simulink model "PI_PSO"  (R2021a)
settings: Solver=VariableStepAuto  StartTime=0.0  StopTime=100  RelTol=1e-6  AbsTol=1e-6
undefined symbols (not defined in the file or in its folder): DiscIntNeverNeededParam, G, Solar_time, wind, wind_time
libraries: powerlib_extras x24, pid_lib x6, simulink x2
(part 1 of 2)
settings Model: Creator=hp  LastModifiedBy=hp
settings SolverCC: ZeroCrossAlgorithm=Adaptive
settings DataIOCC: ReturnWorkspaceOutputs=off
settings DebuggingCC: IgnoredZcDiagnostic=none  SFMachineParentedDataDiag=warning

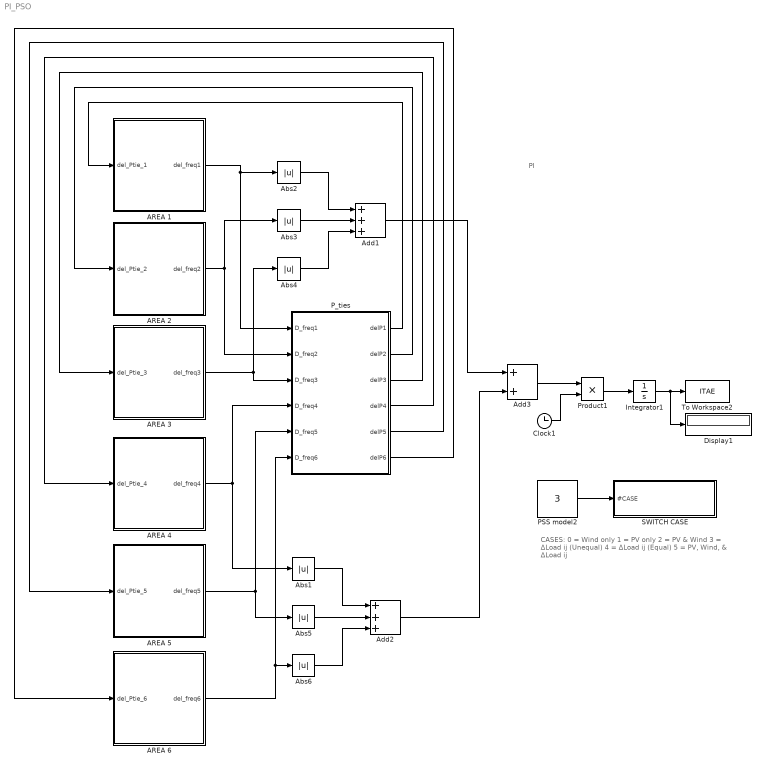
== system PI_PSO ==
  note: PI
  note: CASES:
      |
      | 0 = Wind only
      | 1 = PV only
      | 2 = PV & Wind
      | 3 = ΔLoad ij (Unequal)
      | 4 = ΔLoad ij (Equal)
      | 5 = PV, Wind, & ΔLoad ij
  AREA 1 : Subsystem
  AREA 2 : Subsystem
  AREA 3 : Subsystem
  AREA 4 : Subsystem
  AREA 5 : Subsystem
  AREA 6 : Subsystem
  Abs{1..6} (6 alike) : Abs
  Add1 : Sum  Inputs=+++
  Add2 : Sum  Inputs=+++
  Add3 : Sum
  Clock1 : Clock
  Display1 : Display
  Integrator1 : Integrator
  PSS model2 : Constant  Value=3
  P_ties : Subsystem
  Product1 : Product
  SWITCH CASE : Subsystem
  To Workspace2 : ToWorkspace  VariableName=ITAE  SampleTime=-1
      settings: Save2DSignal=2-D array (concatenate along first dimension)
  wires:
  Abs3/1 -> Add1/2
  AREA 3/1(del_freq3) -> P_ties/3(D_freq3), Abs4/1
  Clock1/1 -> Product1/2
  AREA 1/1(del_freq1) -> P_ties/1(D_freq1), Abs2/1
  AREA 2/1(del_freq2) -> P_ties/2(D_freq2), Abs3/1
  P_ties/2(delP2) -> AREA 2/1(del_Ptie_2)
  Abs4/1 -> Add1/3
  Abs2/1 -> Add1/1
  Add1/1 -> Add3/1
  Product1/1 -> Integrator1/1
  Integrator1/1 -> To Workspace2/1, Display1/1
  P_ties/1(delP1) -> AREA 1/1(del_Ptie_1)
  P_ties/3(delP3) -> AREA 3/1(del_Ptie_3)
  P_ties/4(delP4) -> AREA 4/1(del_Ptie_4)
  P_ties/5(delP5) -> AREA 5/1(del_Ptie_5)
  P_ties/6(delP6) -> AREA 6/1(del_Ptie_6)
  AREA 4/1(del_freq4) -> P_ties/4(D_freq4), Abs1/1
  AREA 5/1(del_freq5) -> P_ties/5(D_freq5), Abs5/1
  AREA 6/1(del_freq6) -> P_ties/6(D_freq6), Abs6/1
  Abs6/1 -> Add2/3
  Abs1/1 -> Add2/1
  Abs5/1 -> Add2/2
  Add2/1 -> Add3/2
  Add3/1 -> Product1/1
  PSS model2/1 -> SWITCH CASE/1(#CASE)

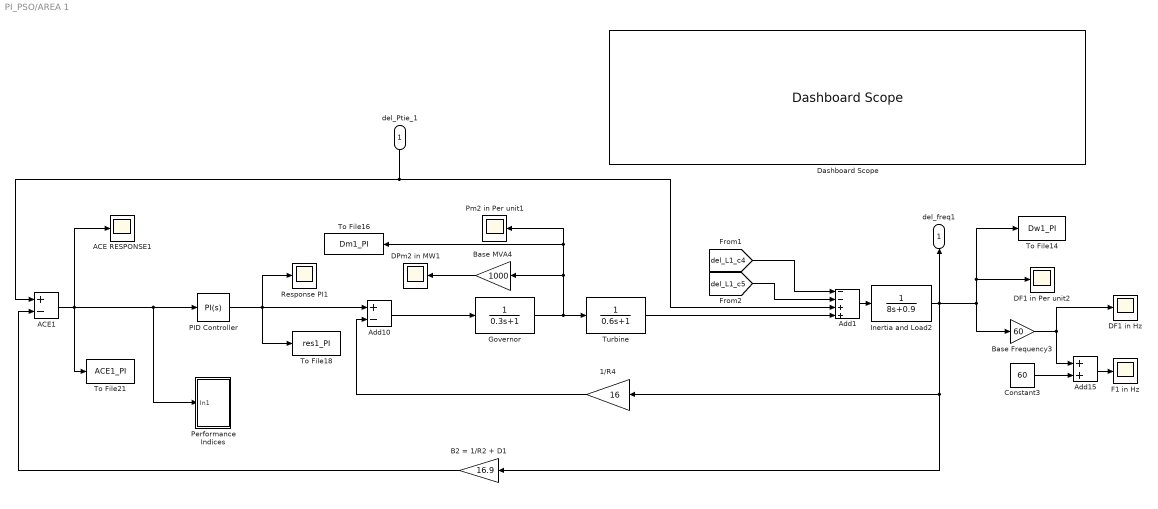
== system PI_PSO/AREA 1 ==
  del_Ptie_1 : Inport
  1/R4 : Gain  Gain=16
  ACE RESPONSE1 : Scope
  ACE1 : Sum  Inputs=+-
  Add1 : Sum  Inputs=--++
  Add10 : Sum  Inputs=+-
  Add15 : Sum
  B2 = 1/R2 + D1 : Gain  Gain=16.9
  Base Frequency3 : Gain  Gain=60
  Base MVA4 : Gain  Gain=1000
  Constant3 : Constant  Value=60
  DF1 in Hz : Scope
  DF1 in Per unit2 : Scope
  DPm2 in MW1 : Scope
  Dashboard Scope : DashboardScope
  F1 in Hz : Scope
  "Governor " : TransferFcn  Denominator=[0.3 1]
  Inertia and Load2 : TransferFcn  Denominator=[8 0.9]
  PID Controller : pid_lib/PID Controller  Controller=PI  Form=Parallel  TimeDomain=Continuous-time  UseExternalTs=off  SampleTime=-1  IntegratorMethod=Forward Euler  FilterMethod=Forward Euler  ControllerParametersSource=internal  P=0.079972086154635  I=0.218754323639510  D=0  UseFilter=on  N=100  TunerSelectOption=Transfer Function Based (PID Tuner App)  InitialConditionSource=internal  InitialConditionForIntegrator=0  InitialConditionForFilter=0  DifferentiatorICPrevScaledInput=0  ExternalReset=none  TrackingMode=off  Kt=1  LimitOutput=off  SatLimitsSource=internal  UpperSaturationLimit=inf  LowerSaturationLimit=-inf  LinearizeAsGain=on  AntiWindupMode=none  Kb=1  POutMin=[]  POutMax=[]  IOutMin=[]  IOutMax=[]  DOutMin=[]  DOutMax=[]  NOutMin=[]  NOutMax=[]  SumOutMin=[]  SumOutMax=[]  SaturationOutMin=[]  SaturationOutMax=[]  PParamMin=[]  PParamMax=[]  IParamMin=[]  IParamMax=[]  DParamMin=[]  DParamMax=[]  NParamMin=[]  NParamMax=[]  KbParamMin=[]  KbParamMax=[]  KtParamMin=[]  KtParamMax=[]  KbOutMin=[]  KbOutMax=[]  KtOutMin=[]  KtOutMax=[]  IntegratorOutMin=[]  IntegratorOutMax=[]  FilterOutMin=[]  FilterOutMax=[]  SumI1OutMin=[]  SumI1OutMax=[]  SumI2OutMin=[]  SumI2OutMax=[]  SumI3OutMin=[]  SumI3OutMax=[]  SumI4OutMin=[]  SumI4OutMax=[]  SumDOutMin=[]  SumDOutMax=[]  DifferentiatorOutMin=[]  DifferentiatorOutMax=[]  FilterDiffOutCoefMin=[]  FilterDiffOutCoefMax=[]  ReciprocalOutMin=[]  ReciprocalOutMax=[]  SumDenOutMin=[]  SumDenOutMax=[]  SumNumOutMin=[]  SumNumOutMax=[]  DivideOutMin=[]  DivideOutMax=[]  UdiffTsProdOutMin=[]  UdiffTsProdOutMax=[]  NTsProdOutMin=[]  NTsProdOutMax=[]  UintegralTsProdOutMin=[]  UintegralTsProdOutMax=[]  UngainTsProdOutMin=[]  UngainTsProdOutMax=[]  IntegratorContinuousStateAttributes=''  IntegratorStateMustResolveToSignalObject=off  IntegratorRTWStateStorageClass=Auto  FilterContinuousStateAttributes=''  FilterStateMustResolveToSignalObject=off  FilterRTWStateStorageClass=Auto  ParallelPVariant=InternalParameters  IdealPVariant=Disabled  IVariant=InternalParameters  DVariant=Disabled  IntegratorVariant=Continuous  SatVariant=Disabled  AWVariant=Passthrough  PCopyVariant=Disabled  TRVariant=Disabled  FdbkBlocksVariant=Forward  IdealPFdbkVariant=Disabled  SatFdbkVariant=Disabled  DerivativeFilterVariant=Disabled  NVariant=Disabled  NCopyVariant=Disabled_SignalSpec  FilterICVariant=Disabled  IntegratorICVariant=InternalICs  ExternalResetVariant=Disabled  TRSumVariant=Passthrough  SumFdbkVariant=Disabled  SumVariant=Sum_PI  TsampFilterVariant=InternalTs  TsampNgainVariant=Passthrough  TsampIntegralVariant=Passthrough  ExternalSaturationOutDataTypeStr=Inherit: Same as second input
  Performance Indices : Subsystem
  Pm2 in Per unit1 : Scope
  Response PI1 : Scope
  To File14 : ToFile  Filename=Dw1_PI  MatrixName=Dw1_PI
  To File16 : ToFile  Filename=Dm1_PI  MatrixName=Dm1_PI
  To File18 : ToFile  Filename=res1_PI  MatrixName=res1_PI
  To File21 : ToFile  Filename=ACE1_PI  MatrixName=ACE1_PI
  Turbine : TransferFcn  Denominator=[0.6 1]
  del_freq1 : Outport
  wires:
  PID Controller/1 -> Response PI1/1, Add10/1, To File18/1
  1/R4/1 -> Add10/2
  Base MVA4/1 -> DPm2 in MW1/1
  Constant3/1 -> Add15/2
  Add15/1 -> F1 in Hz/1
  Base Frequency3/1 -> DF1 in Hz/1, Add15/1
  B2 = 1/R2 + D1/1 -> ACE1/2
  del_Ptie_1/1 -> Add1/3, ACE1/1
  Inertia and Load2/1 -> Base Frequency3/1, To File14/1, DF1 in Per unit2/1, 1/R4/1, B2 = 1/R2 + D1/1, del_freq1/1
  Add1/1 -> Inertia and Load2/1
  ACE1/1 -> PID Controller/1, Performance Indices/1(In1), To File21/1, ACE RESPONSE1/1
  Turbine/1 -> Add1/4
  [del_L1_c4] -> Add1/1
  [del_L1_c5] -> Add1/2
  "Governor "/1 -> Turbine/1, Pm2 in Per unit1/1, To File16/1, Base MVA4/1
  Add10/1 -> "Governor "/1

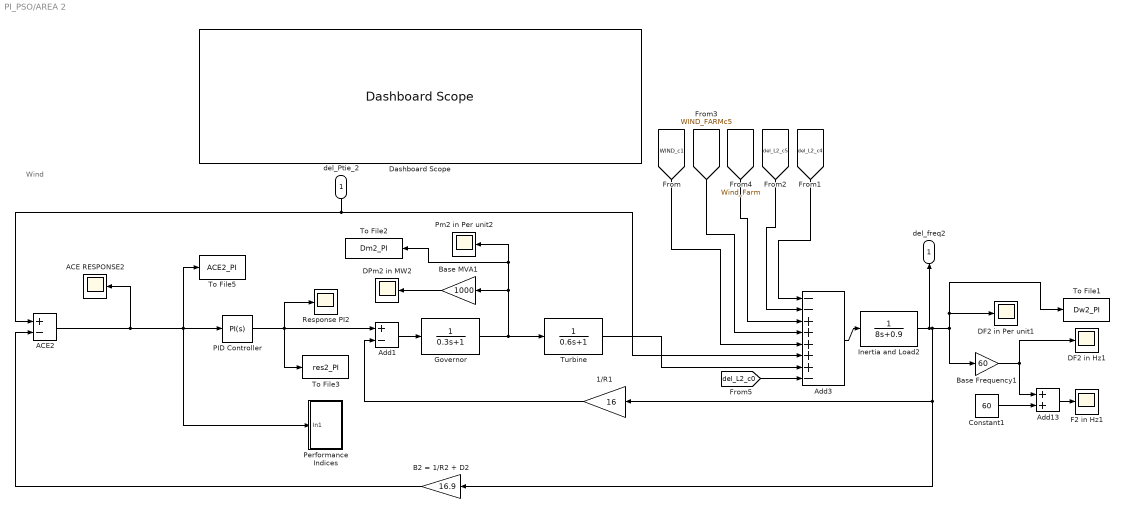
== system PI_PSO/AREA 2 ==
  note: Wind
  del_Ptie_2 : Inport
  1/R1 : Gain  Gain=16
  ACE RESPONSE2 : Scope
  ACE2 : Sum  Inputs=+-
  Add1 : Sum  Inputs=+-
  Add13 : Sum
  Add3 : Sum  Inputs=--+++++-
  B2 = 1/R2 + D2 : Gain  Gain=16.9
  Base Frequency1 : Gain  Gain=60
  Base MVA1 : Gain  Gain=1000
  Constant1 : Constant  Value=60
  DF2 in Hz1 : Scope
  DF2 in Per unit1 : Scope
  DPm2 in MW2 : Scope
  Dashboard Scope : DashboardScope
  F2 in Hz1 : Scope
  "Governor " : TransferFcn  Denominator=[0.3 1]
  Inertia and Load2 : TransferFcn  Denominator=[8 0.9]
  PID Controller : pid_lib/PID Controller  Controller=PI  Form=Parallel  TimeDomain=Continuous-time  UseExternalTs=off  SampleTime=-1  IntegratorMethod=Forward Euler  FilterMethod=Forward Euler  ControllerParametersSource=internal  P=-0.193992496547051  I=0.445472440969199  D=0  UseFilter=on  N=100  TunerSelectOption=Transfer Function Based (PID Tuner App)  InitialConditionSource=internal  InitialConditionForIntegrator=0  InitialConditionForFilter=0  DifferentiatorICPrevScaledInput=0  ExternalReset=none  TrackingMode=off  Kt=1  LimitOutput=off  SatLimitsSource=internal  UpperSaturationLimit=inf  LowerSaturationLimit=-inf  LinearizeAsGain=on  AntiWindupMode=none  Kb=1  POutMin=[]  POutMax=[]  IOutMin=[]  IOutMax=[]  DOutMin=[]  DOutMax=[]  NOutMin=[]  NOutMax=[]  SumOutMin=[]  SumOutMax=[]  SaturationOutMin=[]  SaturationOutMax=[]  PParamMin=[]  PParamMax=[]  IParamMin=[]  IParamMax=[]  DParamMin=[]  DParamMax=[]  NParamMin=[]  NParamMax=[]  KbParamMin=[]  KbParamMax=[]  KtParamMin=[]  KtParamMax=[]  KbOutMin=[]  KbOutMax=[]  KtOutMin=[]  KtOutMax=[]  IntegratorOutMin=[]  IntegratorOutMax=[]  FilterOutMin=[]  FilterOutMax=[]  SumI1OutMin=[]  SumI1OutMax=[]  SumI2OutMin=[]  SumI2OutMax=[]  SumI3OutMin=[]  SumI3OutMax=[]  SumI4OutMin=[]  SumI4OutMax=[]  SumDOutMin=[]  SumDOutMax=[]  DifferentiatorOutMin=[]  DifferentiatorOutMax=[]  FilterDiffOutCoefMin=[]  FilterDiffOutCoefMax=[]  ReciprocalOutMin=[]  ReciprocalOutMax=[]  SumDenOutMin=[]  SumDenOutMax=[]  SumNumOutMin=[]  SumNumOutMax=[]  DivideOutMin=[]  DivideOutMax=[]  UdiffTsProdOutMin=[]  UdiffTsProdOutMax=[]  NTsProdOutMin=[]  NTsProdOutMax=[]  UintegralTsProdOutMin=[]  UintegralTsProdOutMax=[]  UngainTsProdOutMin=[]  UngainTsProdOutMax=[]  IntegratorContinuousStateAttributes=''  IntegratorStateMustResolveToSignalObject=off  IntegratorRTWStateStorageClass=Auto  FilterContinuousStateAttributes=''  FilterStateMustResolveToSignalObject=off  FilterRTWStateStorageClass=Auto  ParallelPVariant=InternalParameters  IdealPVariant=Disabled  IVariant=InternalParameters  DVariant=Disabled  IntegratorVariant=Continuous  SatVariant=Disabled  AWVariant=Passthrough  PCopyVariant=Disabled  TRVariant=Disabled  FdbkBlocksVariant=Forward  IdealPFdbkVariant=Disabled  SatFdbkVariant=Disabled  DerivativeFilterVariant=Disabled  NVariant=Disabled  NCopyVariant=Disabled_SignalSpec  FilterICVariant=Disabled  IntegratorICVariant=InternalICs  ExternalResetVariant=Disabled  TRSumVariant=Passthrough  SumFdbkVariant=Disabled  SumVariant=Sum_PI  TsampFilterVariant=InternalTs  TsampNgainVariant=Passthrough  TsampIntegralVariant=Passthrough  ExternalSaturationOutDataTypeStr=Inherit: Same as second input
  Performance Indices : Subsystem
  Pm2 in Per unit2 : Scope
  Response PI2 : Scope
  To File1 : ToFile  Filename=Dw2_PI  MatrixName=Dw2_PI
  To File2 : ToFile  Filename=Dm2_PI  MatrixName=Dm2_PI
  To File3 : ToFile  Filename=res2_PI  MatrixName=res2_PI
  To File5 : ToFile  Filename=ACE2_PI  MatrixName=ACE2_PI
  Turbine : TransferFcn  Denominator=[0.6 1]
  del_freq2 : Outport
  wires:
  del_Ptie_2/1 -> Add3/6, ACE2/1
  Inertia and Load2/1 -> Base Frequency1/1, To File1/1, DF2 in Per unit1/1, 1/R1/1, B2 = 1/R2 + D2/1, del_freq2/1
  Add13/1 -> F2 in Hz1/1
  Add3/1 -> Inertia and Load2/1
  1/R1/1 -> Add1/2
  Base Frequency1/1 -> DF2 in Hz1/1, Add13/1
  Base MVA1/1 -> DPm2 in MW2/1
  B2 = 1/R2 + D2/1 -> ACE2/2
  PID Controller/1 -> To File3/1, Response PI2/1, Add1/1
  Constant1/1 -> Add13/2
  ACE2/1 -> ACE RESPONSE2/1, PID Controller/1, Performance Indices/1(In1), To File5/1
  Turbine/1 -> Add3/7
  [WIND_c1] -> Add3/5
  [WIND_FARMc5] -> Add3/4
  [Wind_Farm] -> Add3/3
  [del_L2_c5] -> Add3/2
  [del_L2_c4] -> Add3/1
  "Governor "/1 -> Turbine/1, Pm2 in Per unit2/1, To File2/1, Base MVA1/1
  Add1/1 -> "Governor "/1
  [del_L2_c0] -> Add3/8

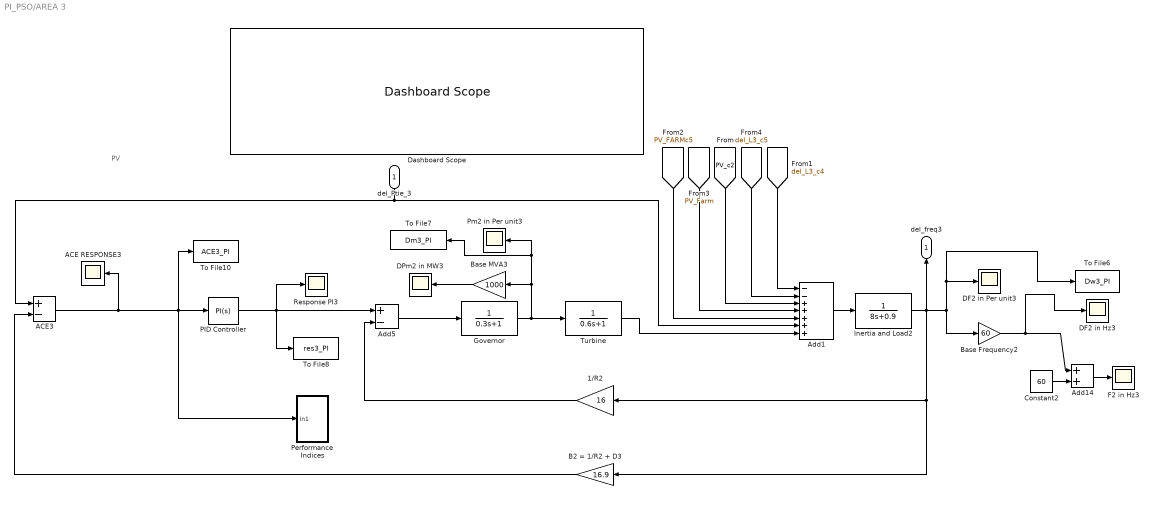
== system PI_PSO/AREA 3 ==
  note: PV
  del_Ptie_3 : Inport
  1/R2 : Gain  Gain=16
  ACE RESPONSE3 : Scope
  ACE3 : Sum  Inputs=+-
  Add1 : Sum  Inputs=--+++++
  Add14 : Sum
  Add5 : Sum  Inputs=+-
  B2 = 1/R2 + D3 : Gain  Gain=16.9
  Base Frequency2 : Gain  Gain=60
  Base MVA3 : Gain  Gain=1000
  Constant2 : Constant  Value=60
  DF2 in Hz3 : Scope
  DF2 in Per unit3 : Scope
  DPm2 in MW3 : Scope
  Dashboard Scope : DashboardScope
  F2 in Hz3 : Scope
  "Governor " : TransferFcn  Denominator=[0.3 1]
  Inertia and Load2 : TransferFcn  Denominator=[8 0.9]
  PID Controller : pid_lib/PID Controller  Controller=PI  Form=Parallel  TimeDomain=Continuous-time  UseExternalTs=off  SampleTime=-1  IntegratorMethod=Forward Euler  FilterMethod=Forward Euler  ControllerParametersSource=internal  P=-0.208794341045674  I=0.479449973673102  D=0  UseFilter=on  N=100  TunerSelectOption=Transfer Function Based (PID Tuner App)  InitialConditionSource=internal  InitialConditionForIntegrator=0  InitialConditionForFilter=0  DifferentiatorICPrevScaledInput=0  ExternalReset=none  TrackingMode=off  Kt=1  LimitOutput=off  SatLimitsSource=internal  UpperSaturationLimit=inf  LowerSaturationLimit=-inf  LinearizeAsGain=on  AntiWindupMode=none  Kb=1  POutMin=[]  POutMax=[]  IOutMin=[]  IOutMax=[]  DOutMin=[]  DOutMax=[]  NOutMin=[]  NOutMax=[]  SumOutMin=[]  SumOutMax=[]  SaturationOutMin=[]  SaturationOutMax=[]  PParamMin=[]  PParamMax=[]  IParamMin=[]  IParamMax=[]  DParamMin=[]  DParamMax=[]  NParamMin=[]  NParamMax=[]  KbParamMin=[]  KbParamMax=[]  KtParamMin=[]  KtParamMax=[]  KbOutMin=[]  KbOutMax=[]  KtOutMin=[]  KtOutMax=[]  IntegratorOutMin=[]  IntegratorOutMax=[]  FilterOutMin=[]  FilterOutMax=[]  SumI1OutMin=[]  SumI1OutMax=[]  SumI2OutMin=[]  SumI2OutMax=[]  SumI3OutMin=[]  SumI3OutMax=[]  SumI4OutMin=[]  SumI4OutMax=[]  SumDOutMin=[]  SumDOutMax=[]  DifferentiatorOutMin=[]  DifferentiatorOutMax=[]  FilterDiffOutCoefMin=[]  FilterDiffOutCoefMax=[]  ReciprocalOutMin=[]  ReciprocalOutMax=[]  SumDenOutMin=[]  SumDenOutMax=[]  SumNumOutMin=[]  SumNumOutMax=[]  DivideOutMin=[]  DivideOutMax=[]  UdiffTsProdOutMin=[]  UdiffTsProdOutMax=[]  NTsProdOutMin=[]  NTsProdOutMax=[]  UintegralTsProdOutMin=[]  UintegralTsProdOutMax=[]  UngainTsProdOutMin=[]  UngainTsProdOutMax=[]  IntegratorContinuousStateAttributes=''  IntegratorStateMustResolveToSignalObject=off  IntegratorRTWStateStorageClass=Auto  FilterContinuousStateAttributes=''  FilterStateMustResolveToSignalObject=off  FilterRTWStateStorageClass=Auto  ParallelPVariant=InternalParameters  IdealPVariant=Disabled  IVariant=InternalParameters  DVariant=Disabled  IntegratorVariant=Continuous  SatVariant=Disabled  AWVariant=Passthrough  PCopyVariant=Disabled  TRVariant=Disabled  FdbkBlocksVariant=Forward  IdealPFdbkVariant=Disabled  SatFdbkVariant=Disabled  DerivativeFilterVariant=Disabled  NVariant=Disabled  NCopyVariant=Disabled_SignalSpec  FilterICVariant=Disabled  IntegratorICVariant=InternalICs  ExternalResetVariant=Disabled  TRSumVariant=Passthrough  SumFdbkVariant=Disabled  SumVariant=Sum_PI  TsampFilterVariant=InternalTs  TsampNgainVariant=Passthrough  TsampIntegralVariant=Passthrough  ExternalSaturationOutDataTypeStr=Inherit: Same as second input
  Performance Indices : Subsystem
  Pm2 in Per unit3 : Scope
  Response PI3 : Scope
  To File10 : ToFile  Filename=ACE3_PI  MatrixName=ACE3_PI
  To File6 : ToFile  Filename=Dw3_PI  MatrixName=Dw3_PI
  To File7 : ToFile  Filename=Dm3_PI  MatrixName=Dm3_PI
  To File8 : ToFile  Filename=res3_PI  MatrixName=res3_PI
  Turbine : TransferFcn  Denominator=[0.6 1]
  del_freq3 : Outport
  wires:
  PID Controller/1 -> To File8/1, Response PI3/1, Add5/1
  Constant2/1 -> Add14/2
  Base MVA3/1 -> DPm2 in MW3/1
  1/R2/1 -> Add5/2
  Base Frequency2/1 -> Add14/1, DF2 in Hz3/1
  Add14/1 -> F2 in Hz3/1
  del_Ptie_3/1 -> ACE3/1, Add1/6
  B2 = 1/R2 + D3/1 -> ACE3/2
  Add1/1 -> Inertia and Load2/1
  Inertia and Load2/1 -> 1/R2/1, B2 = 1/R2 + D3/1, Base Frequency2/1, To File6/1, DF2 in Per unit3/1, del_freq3/1
  ACE3/1 -> ACE RESPONSE3/1, PID Controller/1, Performance Indices/1(In1), To File10/1
  Turbine/1 -> Add1/7
  [PV_FARMc5] -> Add1/5
  [PV_Farm] -> Add1/4
  [PV_c2] -> Add1/3
  [del_L3_c5] -> Add1/2
  [del_L3_c4] -> Add1/1
  Add5/1 -> "Governor "/1
  "Governor "/1 -> Turbine/1, To File7/1, Pm2 in Per unit3/1, Base MVA3/1

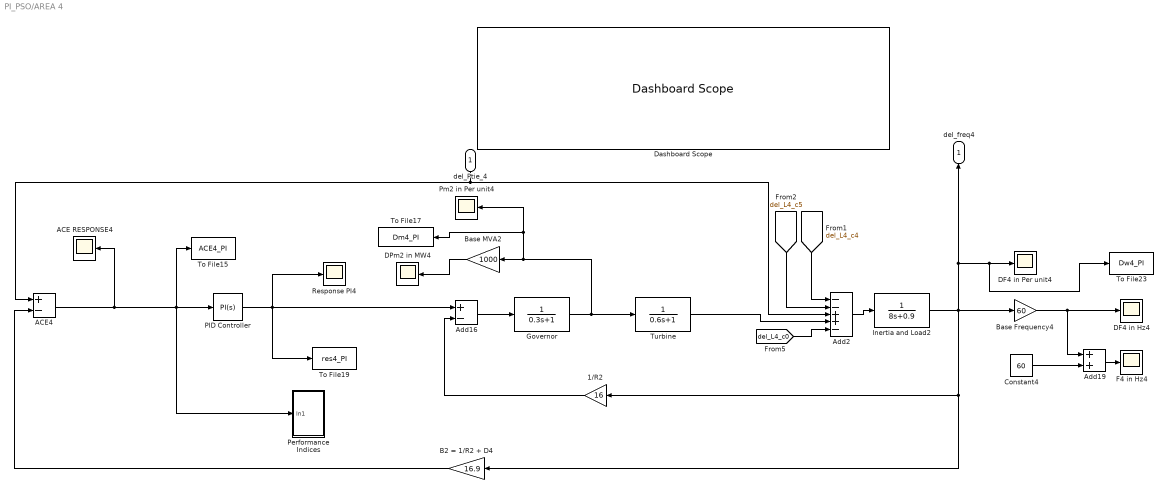
== system PI_PSO/AREA 4 ==
  del_Ptie_4 : Inport
  1/R2 : Gain  Gain=16
  ACE RESPONSE4 : Scope
  ACE4 : Sum  Inputs=+-
  Add16 : Sum  Inputs=+-
  Add19 : Sum
  Add2 : Sum  Inputs=--++-
  B2 = 1/R2 + D4 : Gain  Gain=16.9
  Base Frequency4 : Gain  Gain=60
  Base MVA2 : Gain  Gain=1000
  Constant4 : Constant  Value=60
  DF4 in Hz4 : Scope
  DF4 in Per unit4 : Scope
  DPm2 in MW4 : Scope
  Dashboard Scope : DashboardScope
  F4 in Hz4 : Scope
  "Governor " : TransferFcn  Denominator=[0.3 1]
  Inertia and Load2 : TransferFcn  Denominator=[8 0.9]
  PID Controller : pid_lib/PID Controller  Controller=PI  Form=Parallel  TimeDomain=Continuous-time  UseExternalTs=off  SampleTime=-1  IntegratorMethod=Forward Euler  FilterMethod=Forward Euler  ControllerParametersSource=internal  P=0.085231271598390  I=0.194395137959333  D=0  UseFilter=on  N=100  TunerSelectOption=Transfer Function Based (PID Tuner App)  InitialConditionSource=internal  InitialConditionForIntegrator=0  InitialConditionForFilter=0  DifferentiatorICPrevScaledInput=0  ExternalReset=none  TrackingMode=off  Kt=1  LimitOutput=off  SatLimitsSource=internal  UpperSaturationLimit=inf  LowerSaturationLimit=-inf  LinearizeAsGain=on  AntiWindupMode=none  Kb=1  POutMin=[]  POutMax=[]  IOutMin=[]  IOutMax=[]  DOutMin=[]  DOutMax=[]  NOutMin=[]  NOutMax=[]  SumOutMin=[]  SumOutMax=[]  SaturationOutMin=[]  SaturationOutMax=[]  PParamMin=[]  PParamMax=[]  IParamMin=[]  IParamMax=[]  DParamMin=[]  DParamMax=[]  NParamMin=[]  NParamMax=[]  KbParamMin=[]  KbParamMax=[]  KtParamMin=[]  KtParamMax=[]  KbOutMin=[]  KbOutMax=[]  KtOutMin=[]  KtOutMax=[]  IntegratorOutMin=[]  IntegratorOutMax=[]  FilterOutMin=[]  FilterOutMax=[]  SumI1OutMin=[]  SumI1OutMax=[]  SumI2OutMin=[]  SumI2OutMax=[]  SumI3OutMin=[]  SumI3OutMax=[]  SumI4OutMin=[]  SumI4OutMax=[]  SumDOutMin=[]  SumDOutMax=[]  DifferentiatorOutMin=[]  DifferentiatorOutMax=[]  FilterDiffOutCoefMin=[]  FilterDiffOutCoefMax=[]  ReciprocalOutMin=[]  ReciprocalOutMax=[]  SumDenOutMin=[]  SumDenOutMax=[]  SumNumOutMin=[]  SumNumOutMax=[]  DivideOutMin=[]  DivideOutMax=[]  UdiffTsProdOutMin=[]  UdiffTsProdOutMax=[]  NTsProdOutMin=[]  NTsProdOutMax=[]  UintegralTsProdOutMin=[]  UintegralTsProdOutMax=[]  UngainTsProdOutMin=[]  UngainTsProdOutMax=[]  IntegratorContinuousStateAttributes=''  IntegratorStateMustResolveToSignalObject=off  IntegratorRTWStateStorageClass=Auto  FilterContinuousStateAttributes=''  FilterStateMustResolveToSignalObject=off  FilterRTWStateStorageClass=Auto  ParallelPVariant=InternalParameters  IdealPVariant=Disabled  IVariant=InternalParameters  DVariant=Disabled  IntegratorVariant=Continuous  SatVariant=Disabled  AWVariant=Passthrough  PCopyVariant=Disabled  TRVariant=Disabled  FdbkBlocksVariant=Forward  IdealPFdbkVariant=Disabled  SatFdbkVariant=Disabled  DerivativeFilterVariant=Disabled  NVariant=Disabled  NCopyVariant=Disabled_SignalSpec  FilterICVariant=Disabled  IntegratorICVariant=InternalICs  ExternalResetVariant=Disabled  TRSumVariant=Passthrough  SumFdbkVariant=Disabled  SumVariant=Sum_PI  TsampFilterVariant=InternalTs  TsampNgainVariant=Passthrough  TsampIntegralVariant=Passthrough  ExternalSaturationOutDataTypeStr=Inherit: Same as second input
  Performance Indices : Subsystem
  Pm2 in Per unit4 : Scope
  Response PI4 : Scope
  To File15 : ToFile  Filename=ACE4_PI  MatrixName=ACE4_PI
  To File17 : ToFile  Filename=Dm4_PI  MatrixName=Dm4_PI
  To File19 : ToFile  Filename=res4_PI  MatrixName=res4_PI
  To File23 : ToFile  Filename=Dw4_PI  MatrixName=Dw4_PI
  Turbine : TransferFcn  Denominator=[0.6 1]
  del_freq4 : Outport
  wires:
  ACE4/1 -> ACE RESPONSE4/1, PID Controller/1, Performance Indices/1(In1), To File15/1
  Constant4/1 -> Add19/2
  Add2/1 -> Inertia and Load2/1
  Add19/1 -> F4 in Hz4/1
  B2 = 1/R2 + D4/1 -> ACE4/2
  Base MVA2/1 -> DPm2 in MW4/1
  Inertia and Load2/1 -> B2 = 1/R2 + D4/1, 1/R2/1, Base Frequency4/1, del_freq4/1, To File23/1, DF4 in Per unit4/1
  Base Frequency4/1 -> DF4 in Hz4/1, Add19/1
  1/R2/1 -> Add16/2
  del_Ptie_4/1 -> Add2/3, ACE4/1
  [del_L4_c5] -> Add2/2
  [del_L4_c4] -> Add2/1
  PID Controller/1 -> To File19/1, Response PI4/1, Add16/1
  Add16/1 -> "Governor "/1
  "Governor "/1 -> Turbine/1, To File17/1, Pm2 in Per unit4/1, Base MVA2/1
  Turbine/1 -> Add2/4
  [del_L4_c0] -> Add2/5

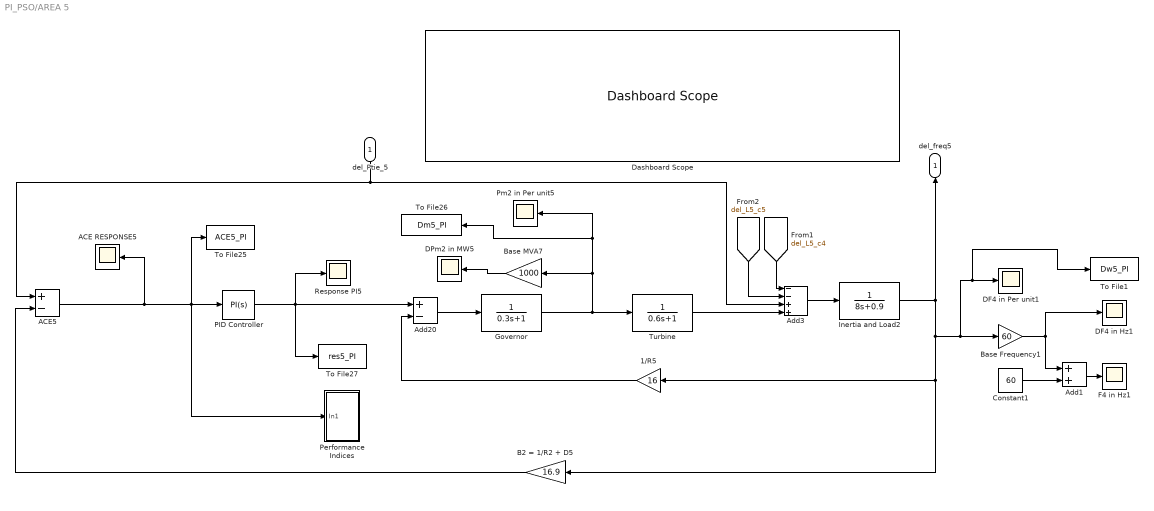
== system PI_PSO/AREA 5 ==
  del_Ptie_5 : Inport
  1/R5 : Gain  Gain=16
  ACE RESPONSE5 : Scope
  ACE5 : Sum  Inputs=+-
  Add1 : Sum
  Add20 : Sum  Inputs=+-
  Add3 : Sum  Inputs=--++
  B2 = 1/R2 + D5 : Gain  Gain=16.9
  Base Frequency1 : Gain  Gain=60
  Base MVA7 : Gain  Gain=1000
  Constant1 : Constant  Value=60
  DF4 in Hz1 : Scope
  DF4 in Per unit1 : Scope
  DPm2 in MW5 : Scope
  Dashboard Scope : DashboardScope
  F4 in Hz1 : Scope
  "Governor " : TransferFcn  Denominator=[0.3 1]
  Inertia and Load2 : TransferFcn  Denominator=[8 0.9]
  PID Controller : pid_lib/PID Controller  Controller=PI  Form=Parallel  TimeDomain=Continuous-time  UseExternalTs=off  SampleTime=-1  IntegratorMethod=Forward Euler  FilterMethod=Forward Euler  ControllerParametersSource=internal  P=-0.426469161483215  I=0.210966324969466  D=0  UseFilter=on  N=100  TunerSelectOption=Transfer Function Based (PID Tuner App)  InitialConditionSource=internal  InitialConditionForIntegrator=0  InitialConditionForFilter=0  DifferentiatorICPrevScaledInput=0  ExternalReset=none  TrackingMode=off  Kt=1  LimitOutput=off  SatLimitsSource=internal  UpperSaturationLimit=inf  LowerSaturationLimit=-inf  LinearizeAsGain=on  AntiWindupMode=none  Kb=1  POutMin=[]  POutMax=[]  IOutMin=[]  IOutMax=[]  DOutMin=[]  DOutMax=[]  NOutMin=[]  NOutMax=[]  SumOutMin=[]  SumOutMax=[]  SaturationOutMin=[]  SaturationOutMax=[]  PParamMin=[]  PParamMax=[]  IParamMin=[]  IParamMax=[]  DParamMin=[]  DParamMax=[]  NParamMin=[]  NParamMax=[]  KbParamMin=[]  KbParamMax=[]  KtParamMin=[]  KtParamMax=[]  KbOutMin=[]  KbOutMax=[]  KtOutMin=[]  KtOutMax=[]  IntegratorOutMin=[]  IntegratorOutMax=[]  FilterOutMin=[]  FilterOutMax=[]  SumI1OutMin=[]  SumI1OutMax=[]  SumI2OutMin=[]  SumI2OutMax=[]  SumI3OutMin=[]  SumI3OutMax=[]  SumI4OutMin=[]  SumI4OutMax=[]  SumDOutMin=[]  SumDOutMax=[]  DifferentiatorOutMin=[]  DifferentiatorOutMax=[]  FilterDiffOutCoefMin=[]  FilterDiffOutCoefMax=[]  ReciprocalOutMin=[]  ReciprocalOutMax=[]  SumDenOutMin=[]  SumDenOutMax=[]  SumNumOutMin=[]  SumNumOutMax=[]  DivideOutMin=[]  DivideOutMax=[]  UdiffTsProdOutMin=[]  UdiffTsProdOutMax=[]  NTsProdOutMin=[]  NTsProdOutMax=[]  UintegralTsProdOutMin=[]  UintegralTsProdOutMax=[]  UngainTsProdOutMin=[]  UngainTsProdOutMax=[]  IntegratorContinuousStateAttributes=''  IntegratorStateMustResolveToSignalObject=off  IntegratorRTWStateStorageClass=Auto  FilterContinuousStateAttributes=''  FilterStateMustResolveToSignalObject=off  FilterRTWStateStorageClass=Auto  ParallelPVariant=InternalParameters  IdealPVariant=Disabled  IVariant=InternalParameters  DVariant=Disabled  IntegratorVariant=Continuous  SatVariant=Disabled  AWVariant=Passthrough  PCopyVariant=Disabled  TRVariant=Disabled  FdbkBlocksVariant=Forward  IdealPFdbkVariant=Disabled  SatFdbkVariant=Disabled  DerivativeFilterVariant=Disabled  NVariant=Disabled  NCopyVariant=Disabled_SignalSpec  FilterICVariant=Disabled  IntegratorICVariant=InternalICs  ExternalResetVariant=Disabled  TRSumVariant=Passthrough  SumFdbkVariant=Disabled  SumVariant=Sum_PI  TsampFilterVariant=InternalTs  TsampNgainVariant=Passthrough  TsampIntegralVariant=Passthrough  ExternalSaturationOutDataTypeStr=Inherit: Same as second input
  Performance Indices : Subsystem
  Pm2 in Per unit5 : Scope
  Response PI5 : Scope
  To File1 : ToFile  Filename=Dw5_PI  MatrixName=Dw5_PI
  To File25 : ToFile  Filename=ACE5_PI  MatrixName=ACE5_PI
  To File26 : ToFile  Filename=Dm5_PI  MatrixName=Dm5_PI
  To File27 : ToFile  Filename=res5_PI  MatrixName=res5_PI
  Turbine : TransferFcn  Denominator=[0.6 1]
  del_freq5 : Outport
  wires:
  Constant1/1 -> Add1/2
  Base MVA7/1 -> DPm2 in MW5/1
  Base Frequency1/1 -> DF4 in Hz1/1, Add1/1
  Add1/1 -> F4 in Hz1/1
  1/R5/1 -> Add20/2
  Add3/1 -> Inertia and Load2/1
  ACE5/1 -> ACE RESPONSE5/1, PID Controller/1, Performance Indices/1(In1), To File25/1
  B2 = 1/R2 + D5/1 -> ACE5/2
  Inertia and Load2/1 -> B2 = 1/R2 + D5/1, 1/R5/1, To File1/1, DF4 in Per unit1/1, Base Frequency1/1, del_freq5/1
  Turbine/1 -> Add3/4
  del_Ptie_5/1 -> ACE5/1, Add3/3
  [del_L5_c5] -> Add3/2
  [del_L5_c4] -> Add3/1
  PID Controller/1 -> To File27/1, Add20/1, Response PI5/1
  Add20/1 -> "Governor "/1
  "Governor "/1 -> To File26/1, Pm2 in Per unit5/1, Base MVA7/1, Turbine/1

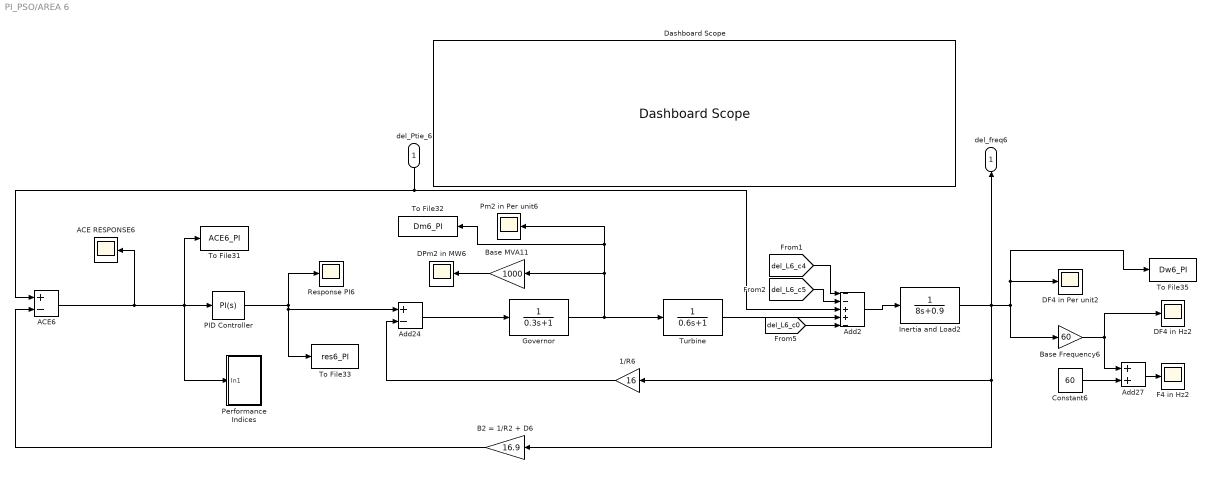
== system PI_PSO/AREA 6 ==
  del_Ptie_6 : Inport
  1/R6 : Gain  Gain=16
  ACE RESPONSE6 : Scope
  ACE6 : Sum  Inputs=+-
  Add2 : Sum  Inputs=--++-
  Add24 : Sum  Inputs=+-
  Add27 : Sum
  B2 = 1/R2 + D6 : Gain  Gain=16.9
  Base Frequency6 : Gain  Gain=60
  Base MVA11 : Gain  Gain=1000
  Constant6 : Constant  Value=60
  DF4 in Hz2 : Scope
  DF4 in Per unit2 : Scope
  DPm2 in MW6 : Scope
  Dashboard Scope : DashboardScope
  F4 in Hz2 : Scope
  "Governor " : TransferFcn  Denominator=[0.3 1]
  Inertia and Load2 : TransferFcn  Denominator=[8 0.9]
  PID Controller : pid_lib/PID Controller  Controller=PI  Form=Parallel  TimeDomain=Continuous-time  UseExternalTs=off  SampleTime=-1  IntegratorMethod=Forward Euler  FilterMethod=Forward Euler  ControllerParametersSource=internal  P=-0.029658962972710  I=0.090847703671048  D=0  UseFilter=on  N=100  TunerSelectOption=Transfer Function Based (PID Tuner App)  InitialConditionSource=internal  InitialConditionForIntegrator=0  InitialConditionForFilter=0  DifferentiatorICPrevScaledInput=0  ExternalReset=none  TrackingMode=off  Kt=1  LimitOutput=off  SatLimitsSource=internal  UpperSaturationLimit=inf  LowerSaturationLimit=-inf  LinearizeAsGain=on  AntiWindupMode=none  Kb=1  POutMin=[]  POutMax=[]  IOutMin=[]  IOutMax=[]  DOutMin=[]  DOutMax=[]  NOutMin=[]  NOutMax=[]  SumOutMin=[]  SumOutMax=[]  SaturationOutMin=[]  SaturationOutMax=[]  PParamMin=[]  PParamMax=[]  IParamMin=[]  IParamMax=[]  DParamMin=[]  DParamMax=[]  NParamMin=[]  NParamMax=[]  KbParamMin=[]  KbParamMax=[]  KtParamMin=[]  KtParamMax=[]  KbOutMin=[]  KbOutMax=[]  KtOutMin=[]  KtOutMax=[]  IntegratorOutMin=[]  IntegratorOutMax=[]  FilterOutMin=[]  FilterOutMax=[]  SumI1OutMin=[]  SumI1OutMax=[]  SumI2OutMin=[]  SumI2OutMax=[]  SumI3OutMin=[]  SumI3OutMax=[]  SumI4OutMin=[]  SumI4OutMax=[]  SumDOutMin=[]  SumDOutMax=[]  DifferentiatorOutMin=[]  DifferentiatorOutMax=[]  FilterDiffOutCoefMin=[]  FilterDiffOutCoefMax=[]  ReciprocalOutMin=[]  ReciprocalOutMax=[]  SumDenOutMin=[]  SumDenOutMax=[]  SumNumOutMin=[]  SumNumOutMax=[]  DivideOutMin=[]  DivideOutMax=[]  UdiffTsProdOutMin=[]  UdiffTsProdOutMax=[]  NTsProdOutMin=[]  NTsProdOutMax=[]  UintegralTsProdOutMin=[]  UintegralTsProdOutMax=[]  UngainTsProdOutMin=[]  UngainTsProdOutMax=[]  IntegratorContinuousStateAttributes=''  IntegratorStateMustResolveToSignalObject=off  IntegratorRTWStateStorageClass=Auto  FilterContinuousStateAttributes=''  FilterStateMustResolveToSignalObject=off  FilterRTWStateStorageClass=Auto  ParallelPVariant=InternalParameters  IdealPVariant=Disabled  IVariant=InternalParameters  DVariant=Disabled  IntegratorVariant=Continuous  SatVariant=Disabled  AWVariant=Passthrough  PCopyVariant=Disabled  TRVariant=Disabled  FdbkBlocksVariant=Forward  IdealPFdbkVariant=Disabled  SatFdbkVariant=Disabled  DerivativeFilterVariant=Disabled  NVariant=Disabled  NCopyVariant=Disabled_SignalSpec  FilterICVariant=Disabled  IntegratorICVariant=InternalICs  ExternalResetVariant=Disabled  TRSumVariant=Passthrough  SumFdbkVariant=Disabled  SumVariant=Sum_PI  TsampFilterVariant=InternalTs  TsampNgainVariant=Passthrough  TsampIntegralVariant=Passthrough  ExternalSaturationOutDataTypeStr=Inherit: Same as second input
  Performance Indices : Subsystem
  Pm2 in Per unit6 : Scope
  Response PI6 : Scope
  To File31 : ToFile  Filename=ACE6_PI  MatrixName=ACE6_PI
  To File32 : ToFile  Filename=Dm6_PI  MatrixName=Dm6_PI
  To File33 : ToFile  Filename=res6_PI  MatrixName=res6_PI
  To File35 : ToFile  Filename=Dw6_PI  MatrixName=Dw6_PI
  Turbine : TransferFcn  Denominator=[0.6 1]
  del_freq6 : Outport
  wires:
  Add27/1 -> F4 in Hz2/1
  B2 = 1/R2 + D6/1 -> ACE6/2
  ACE6/1 -> ACE RESPONSE6/1, PID Controller/1, Performance Indices/1(In1), To File31/1
  1/R6/1 -> Add24/2
  Constant6/1 -> Add27/2
  Base Frequency6/1 -> DF4 in Hz2/1, Add27/1
  Base MVA11/1 -> DPm2 in MW6/1
  Add2/1 -> Inertia and Load2/1
  Inertia and Load2/1 -> B2 = 1/R2 + D6/1, 1/R6/1, del_freq6/1, To File35/1, DF4 in Per unit2/1, Base Frequency6/1
  del_Ptie_6/1 -> Add2/3, ACE6/1
  [del_L6_c4] -> Add2/1
  [del_L6_c5] -> Add2/2
  PID Controller/1 -> Add24/1, To File33/1, Response PI6/1
  Add24/1 -> "Governor "/1
  "Governor "/1 -> Turbine/1, Pm2 in Per unit6/1, To File32/1, Base MVA11/1
  Turbine/1 -> Add2/4
  [del_L6_c0] -> Add2/5

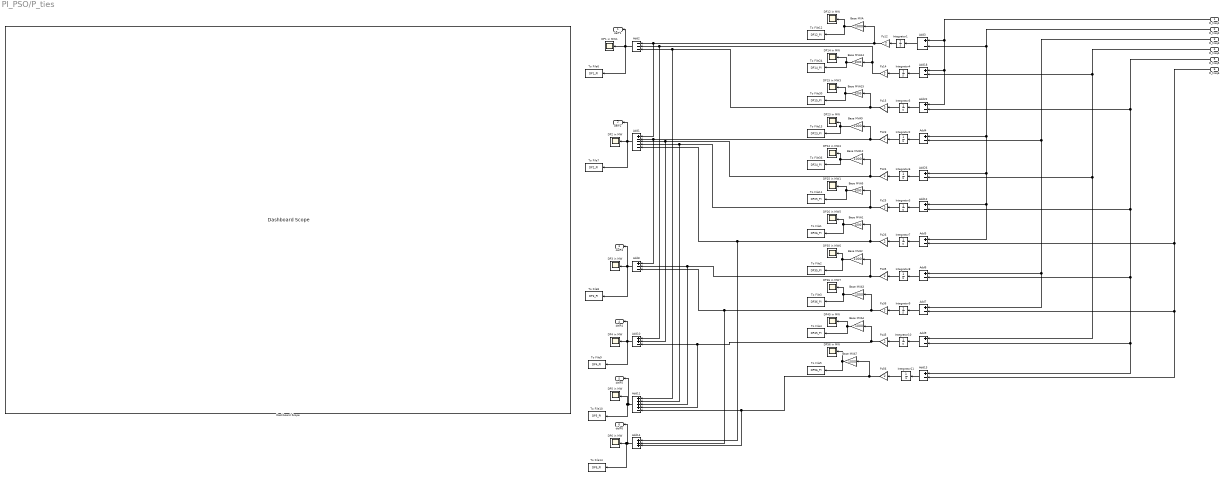
== system PI_PSO/P_ties ==
  D_freq1 : Inport
  D_freq2 : Inport  Port=2
  D_freq3 : Inport  Port=3
  D_freq4 : Inport  Port=4
  D_freq5 : Inport  Port=5
  D_freq6 : Inport  Port=6
  Add1 : Sum  Inputs=+----
  Add10 : Sum  Inputs=++-
  Add11 : Sum  Inputs=++++-
  Add{3..7,9,12..13,18,22,26} (11 alike) : Sum  Inputs=+-
  Add14 : Sum  Inputs=+++
  Add2 : Sum  Inputs=---
  Add8 : Sum  Inputs=+--
  Base MVA{,1..5,7,9,12,14..15} (11 alike) : Gain  Gain=1000
  DP1 in MW1 : Scope
  DP12 in MW : Scope
  DP14 in MW : Scope
  DP15 in MW3 : Scope
  DP2 in MW : Scope
  DP23 in MW : Scope
  DP24 in MW4 : Scope
  DP25 in MW1 : Scope
  DP26 in MW5 : Scope
  DP3 in MW : Scope
  DP35 in MW6 : Scope
  DP36 in MW7 : Scope
  DP4 in MW : Scope
  DP45 in MW : Scope
  DP5 in MW : Scope
  DP56 in MW : Scope
  DP6 in MW : Scope
  Dashboard Scope : DashboardScope
  Integrator{1..11} (11 alike) : Integrator
  Ps{12,14..15,23..26,35..36,45,56} (11 alike) : Gain  Gain=2
  To File1 : ToFile  Filename=DP26_PI  MatrixName=DP26_PI
  To File10 : ToFile  Filename=DP5_PI  MatrixName=DP5_PI
  To File11 : ToFile  Filename=DP25_PI  MatrixName=DP25_PI
  To File12 : ToFile  Filename=DP12_PI  MatrixName=DP12_PI
  To File13 : ToFile  Filename=DP23_PI  MatrixName=DP23_PI
  To File14 : ToFile  Filename=DP6_PI  MatrixName=DP6_PI
  To File2 : ToFile  Filename=DP35_PI  MatrixName=DP35_PI
  To File24 : ToFile  Filename=DP14_PI  MatrixName=DP14_PI
  To File3 : ToFile  Filename=DP36_PI  MatrixName=DP36_PI
  To File30 : ToFile  Filename=DP15_PI  MatrixName=DP15_PI
  To File36 : ToFile  Filename=DP24_PI  MatrixName=DP24_PI
  To File4 : ToFile  Filename=DP45_PI  MatrixName=DP45_PI
  To File5 : ToFile  Filename=DP56_PI  MatrixName=DP56_PI
  To File6 : ToFile  Filename=DP1_PI  MatrixName=DP1_PI
  To File7 : ToFile  Filename=DP2_PI  MatrixName=DP2_PI
  To File8 : ToFile  Filename=DP3_PI  MatrixName=DP3_PI
  To File9 : ToFile  Filename=DP4_PI  MatrixName=DP4_PI
  delP1 : Outport
  delP2 : Outport  Port=2
  delP3 : Outport  Port=3
  delP4 : Outport  Port=4
  delP5 : Outport  Port=5
  delP6 : Outport  Port=6
  wires:
  Add3/1 -> Integrator1/1
  Integrator1/1 -> Ps12/1
  Base MVA/1 -> To File12/1, DP12 in MW/1
  D_freq1/1 -> Add22/1, Add18/1, Add3/1
  D_freq2/1 -> Add5/1, Add12/1, Add26/1, Add4/1, Add3/2
  Integrator4/1 -> Ps14/1
  Add18/1 -> Integrator4/1
  Base MVA14/1 -> To File24/1, DP14 in MW/1
  D_freq4/1 -> Add9/1, Add26/2, Add18/2
  Base MVA15/1 -> To File30/1, DP15 in MW3/1
  Integrator5/1 -> Ps15/1
  Add22/1 -> Integrator5/1
  D_freq5/1 -> Add13/1, Add9/2, Add6/2, Add12/2, Add22/2
  Integrator2/1 -> Ps23/1
  Add4/1 -> Integrator2/1
  Base MVA9/1 -> DP23 in MW/1, To File13/1
  Base MVA12/1 -> DP24 in MW4/1, To File36/1
  Integrator6/1 -> Ps24/1
  Add26/1 -> Integrator6/1
  D_freq3/1 -> Add7/1, Add6/1, Add4/2
  Integrator3/1 -> Ps25/1
  Base MVA5/1 -> To File11/1, DP25 in MW1/1
  Add12/1 -> Integrator3/1
  Add5/1 -> Integrator7/1
  Base MVA1/1 -> To File1/1, DP26 in MW5/1
  Integrator7/1 -> Ps26/1
  D_freq6/1 -> Add13/2, Add7/2, Add5/2
  Base MVA2/1 -> To File2/1, DP35 in MW6/1
  Integrator8/1 -> Ps35/1
  Add6/1 -> Integrator8/1
  Add7/1 -> Integrator9/1
  Base MVA3/1 -> To File3/1, DP36 in MW7/1
  Integrator9/1 -> Ps36/1
  Add9/1 -> Integrator10/1
  Integrator10/1 -> Ps45/1
  Base MVA4/1 -> DP45 in MW/1, To File4/1
  Integrator11/1 -> Ps56/1
  Add13/1 -> Integrator11/1
  Base MVA7/1 -> DP56 in MW/1, To File5/1
  Ps24/1 -> Add10/2, Add1/3, Base MVA12/1
  Ps15/1 -> Add11/1, Add2/3, Base MVA15/1
  Ps12/1 -> Base MVA/1, Add1/1, Add2/1
  Ps35/1 -> Add11/3, Add8/2, Base MVA2/1
  Ps23/1 -> Add8/1, Add1/2, Base MVA9/1
  Ps56/1 -> Base MVA7/1, Add14/3, Add11/5
  Ps26/1 -> Add14/1, Add1/5, Base MVA1/1
  Ps14/1 -> Add10/1, Add2/2, Base MVA14/1
  Ps25/1 -> Add11/2, Add1/4, Base MVA5/1
  Ps36/1 -> Add14/2, Add8/3, Base MVA3/1
  Ps45/1 -> Add11/4, Add10/3, Base MVA4/1
  Add2/1 -> To File6/1, delP1/1, DP1 in MW1/1
  Add1/1 -> To File7/1, DP2 in MW/1, delP2/1
  Add8/1 -> delP3/1, To File8/1, DP3 in MW/1
  Add10/1 -> To File9/1, delP4/1, DP4 in MW/1
  Add11/1 -> delP5/1, To File10/1, DP5 in MW/1
  Add14/1 -> delP6/1, To File14/1, DP6 in MW/1

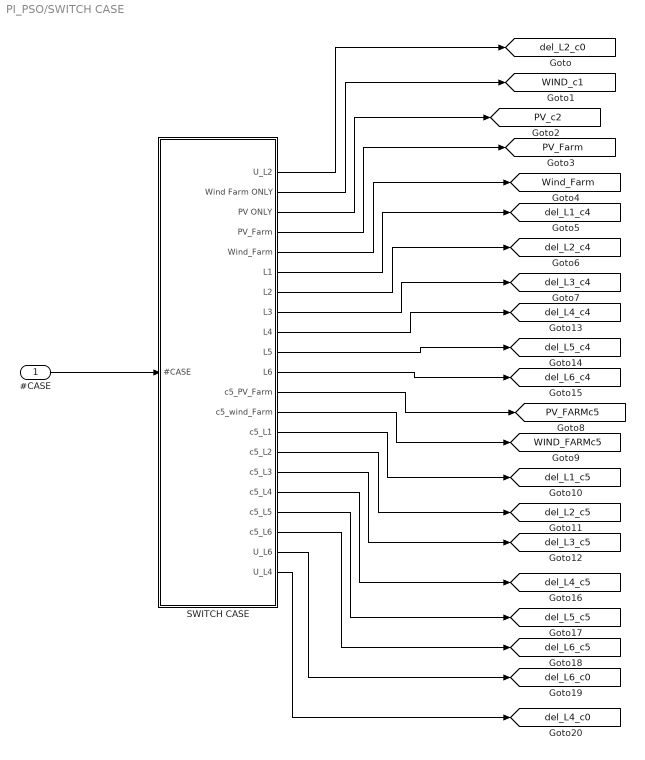
== system PI_PSO/SWITCH CASE ==
  #CASE : Inport
  SWITCH CASE : Subsystem
  tag scope: PV_FARMc5=global, PV_Farm=global, PV_c2=global, WIND_FARMc5=global, WIND_c1=global, Wind_Farm=global, del_L1_c4=global, del_L1_c5=global, del_L2_c0=global, del_L2_c4=global, del_L2_c5=global, del_L3_c4=global, del_L3_c5=global, del_L4_c0=global, del_L4_c4=global, del_L4_c5=global, del_L5_c4=global, del_L5_c5=global, del_L6_c0=global, del_L6_c4=global, del_L6_c5=global
  wires:
  SWITCH CASE/9("L4 ") -> [del_L4_c4]
  SWITCH CASE/15(c5_L2) -> [del_L2_c5]
  SWITCH CASE/10("L5 ") -> [del_L5_c4]
  SWITCH CASE/11("L6 ") -> [del_L6_c4]
  SWITCH CASE/1(U_L2) -> [del_L2_c0]
  #CASE/1 -> SWITCH CASE/1(#CASE)
  SWITCH CASE/12(c5_PV_Farm) -> [PV_FARMc5]
  SWITCH CASE/14(c5_L1) -> [del_L1_c5]
  SWITCH CASE/3("PV ONLY ") -> [PV_c2]
  SWITCH CASE/6("L1 ") -> [del_L1_c4]
  SWITCH CASE/4("PV_Farm ") -> [PV_Farm]
  SWITCH CASE/13(c5_wind_Farm) -> [WIND_FARMc5]
  SWITCH CASE/7("L2 ") -> [del_L2_c4]
  SWITCH CASE/2("Wind Farm ONLY ") -> [WIND_c1]
  SWITCH CASE/16("c5_L3 ") -> [del_L3_c5]
  SWITCH CASE/8("L3 ") -> [del_L3_c4]
  SWITCH CASE/5("Wind_Farm ") -> [Wind_Farm]
  SWITCH CASE/17(c5_L4) -> [del_L4_c5]
  SWITCH CASE/18(c5_L5) -> [del_L5_c5]
  SWITCH CASE/19(c5_L6) -> [del_L6_c5]
  SWITCH CASE/20(U_L6) -> [del_L6_c0]
  SWITCH CASE/21(U_L4) -> [del_L4_c0]

== system PI_PSO/AREA 1/Performance Indices ==
  In1 : Inport
  IAE : Subsystem
      mask help:
      | IAE performacne index
      |
      | output = int |input| dt
      mask Display:
      | disp('IAE')
      | port_label('input',1,'e')
      | port_label('output',1,'iae')
  ISE : Subsystem
      mask help:
      | ISE performance index
      |
      | output = int (input)^2 dt
      mask Display:
      | disp('ISE')
      | port_label('input',1,'e')
      | port_label('output',1,'ise')
  ITAE1 : Subsystem
      mask help:
      | ITAE performance index
      |
      | output = int t|input| dt
      mask Display:
      | disp('ITAE')
      | port_label('input',1,'e')
      | port_label('output',1,'itae')
  ITSE : Subsystem
      mask help:
      | ITAE performance index
      |
      | output = int t|input| dt
      mask Display:
      | disp('ITSE')
      | port_label('input',1,'e')
      | port_label('output',1,'itse')
  Subsystem1 : Subsystem
  Subsystem2 : Subsystem
  Subsystem4 : Subsystem
  Subsystem5 : Subsystem
  To File20 : ToFile  Filename=ITAE_ACE_PI_1  MatrixName=ITAE_ACE_PI_1
  To File27 : ToFile  Filename=IAE_ACE_PI_1  MatrixName=IAE_ACE_PI_1
  To File29 : ToFile  Filename=ISE_ACE_PI_1  MatrixName=ISE_ACE_PI_1
  To File30 : ToFile  Filename=ITSE_ACE_PI_1  MatrixName=ITSE_ACE_PI_1
  wires:
  Subsystem2/1(Out1) -> To File27/1
  In1/1 -> IAE/1(In1), ITSE/1(In1), ISE/1(In1), ITAE1/1(In1)
  Subsystem1/1(Out1) -> To File29/1
  Subsystem5/1(Out1) -> To File30/1
  ISE/1(Out1) -> Subsystem1/1(In1)
  Subsystem4/1(DP1) -> To File20/1
  IAE/1(Out1) -> Subsystem2/1(In1)
  ITAE1/1(Out1) -> Subsystem4/1(In1)
  ITSE/1(Out1) -> Subsystem5/1(In1)

== system PI_PSO/AREA 2/Performance Indices ==
  In1 : Inport
  IAE : Subsystem
      mask help:
      | IAE performacne index
      |
      | output = int |input| dt
      mask Display:
      | disp('IAE')
      | port_label('input',1,'e')
      | port_label('output',1,'iae')
  ISE : Subsystem
      mask help:
      | ISE performance index
      |
      | output = int (input)^2 dt
      mask Display:
      | disp('ISE')
      | port_label('input',1,'e')
      | port_label('output',1,'ise')
  ITAE1 : Subsystem
      mask help:
      | ITAE performance index
      |
      | output = int t|input| dt
      mask Display:
      | disp('ITAE')
      | port_label('input',1,'e')
      | port_label('output',1,'itae')
  ITSE : Subsystem
      mask help:
      | ITAE performance index
      |
      | output = int t|input| dt
      mask Display:
      | disp('ITSE')
      | port_label('input',1,'e')
      | port_label('output',1,'itse')
  Subsystem1 : Subsystem
  Subsystem2 : Subsystem
  Subsystem3 : Subsystem
  Subsystem5 : Subsystem
  To File27 : ToFile  Filename=IAE_ACE_PI_2  MatrixName=IAE_ACE_PI_2
  To File29 : ToFile  Filename=ISE_ACE_PI_2  MatrixName=ISE_ACE_PI_2
  To File30 : ToFile  Filename=ITSE_ACE_PI_2  MatrixName=ITSE_ACE_PI_2
  To File4 : ToFile  Filename=ITAE_ACE_PI_2  MatrixName=ITAE_ACE_PI_2
  wires:
  ITSE/1(Out1) -> Subsystem5/1(In1)
  Subsystem3/1(Out1) -> To File27/1
  In1/1 -> IAE/1(In1), ITSE/1(In1), ISE/1(In1), ITAE1/1(In1)
  IAE/1(Out1) -> Subsystem3/1(In1)
  Subsystem2/1(Out1) -> To File29/1
  ITAE1/1(Out1) -> Subsystem1/1(In1)
  Subsystem1/1(DP1) -> To File4/1
  ISE/1(Out1) -> Subsystem2/1(In1)
  Subsystem5/1(Out1) -> To File30/1

== system PI_PSO/AREA 3/Performance Indices ==
  In1 : Inport
  IAE : Subsystem
      mask help:
      | IAE performacne index
      |
      | output = int |input| dt
      mask Display:
      | disp('IAE')
      | port_label('input',1,'e')
      | port_label('output',1,'iae')
  ISE : Subsystem
      mask help:
      | ISE performance index
      |
      | output = int (input)^2 dt
      mask Display:
      | disp('ISE')
      | port_label('input',1,'e')
      | port_label('output',1,'ise')
  ITAE2 : Subsystem
      mask help:
      | ITAE performance index
      |
      | output = int t|input| dt
      mask Display:
      | disp('ITAE')
      | port_label('input',1,'e')
      | port_label('output',1,'itae')
  ITSE : Subsystem
      mask help:
      | ITAE performance index
      |
      | output = int t|input| dt
      mask Display:
      | disp('ITSE')
      | port_label('input',1,'e')
      | port_label('output',1,'itse')
  Subsystem1 : Subsystem
  Subsystem2 : Subsystem
  Subsystem3 : Subsystem
  Subsystem5 : Subsystem
  To File27 : ToFile  Filename=IAE_ACE_PI_3  MatrixName=IAE_ACE_PI_3
  To File29 : ToFile  Filename=ISE_ACE_PI_3  MatrixName=ISE_ACE_PI_3
  To File30 : ToFile  Filename=ITSE_ACE_PI_3  MatrixName=ITSE_ACE_PI_3
  To File9 : ToFile  Filename=ITAE_ACE_PI_3  MatrixName=ITAE_ACE_PI_3
  wires:
  In1/1 -> IAE/1(In1), ISE/1(In1), ITSE/1(In1), ITAE2/1(In1)
  ISE/1(Out1) -> Subsystem1/1(In1)
  ITSE/1(Out1) -> Subsystem5/1(In1)
  Subsystem2/1(DP1) -> To File9/1
  ITAE2/1(Out1) -> Subsystem2/1(In1)
  Subsystem3/1(Out1) -> To File27/1
  Subsystem1/1(Out1) -> To File29/1
  IAE/1(Out1) -> Subsystem3/1(In1)
  Subsystem5/1(Out1) -> To File30/1

== system PI_PSO/AREA 4/Performance Indices ==
  In1 : Inport
  IAE : Subsystem
      mask help:
      | IAE performacne index
      |
      | output = int |input| dt
      mask Display:
      | disp('IAE')
      | port_label('input',1,'e')
      | port_label('output',1,'iae')
  ISE : Subsystem
      mask help:
      | ISE performance index
      |
      | output = int (input)^2 dt
      mask Display:
      | disp('ISE')
      | port_label('input',1,'e')
      | port_label('output',1,'ise')
  ITAE4 : Subsystem
      mask help:
      | ITAE performance index
      |
      | output = int t|input| dt
      mask Display:
      | disp('ITAE')
      | port_label('input',1,'e')
      | port_label('output',1,'itae')
  ITSE : Subsystem
      mask help:
      | ITAE performance index
      |
      | output = int t|input| dt
      mask Display:
      | disp('ITSE')
      | port_label('input',1,'e')
      | port_label('output',1,'itse')
  Subsystem1 : Subsystem
  Subsystem2 : Subsystem
  Subsystem3 : Subsystem
  Subsystem5 : Subsystem
  To File22 : ToFile  Filename=ITAE_ACE_PI_4  MatrixName=ITAE_ACE_PI_4
  To File27 : ToFile  Filename=IAE_ACE_PI_4  MatrixName=IAE_ACE_PI_4
  To File29 : ToFile  Filename=ISE_ACE_PI_4  MatrixName=ISE_ACE_PI_4
  To File30 : ToFile  Filename=ITSE_ACE_PI_4  MatrixName=ITSE_ACE_PI_4
  wires:
  ITAE4/1(Out1) -> Subsystem3/1(In1)
  IAE/1(Out1) -> Subsystem2/1(In1)
  Subsystem2/1(Out1) -> To File27/1
  ITSE/1(Out1) -> Subsystem5/1(In1)
  Subsystem1/1(Out1) -> To File29/1
  In1/1 -> ITSE/1(In1), ISE/1(In1), IAE/1(In1), ITAE4/1(In1)
  Subsystem5/1(Out1) -> To File30/1
  Subsystem3/1(DP1) -> To File22/1
  ISE/1(Out1) -> Subsystem1/1(In1)

== system PI_PSO/AREA 5/Performance Indices ==
  In1 : Inport
  IAE : Subsystem
      mask help:
      | IAE performacne index
      |
      | output = int |input| dt
      mask Display:
      | disp('IAE')
      | port_label('input',1,'e')
      | port_label('output',1,'iae')
  ISE : Subsystem
      mask help:
      | ISE performance index
      |
      | output = int (input)^2 dt
      mask Display:
      | disp('ISE')
      | port_label('input',1,'e')
      | port_label('output',1,'ise')
  ITAE5 : Subsystem
      mask help:
      | ITAE performance index
      |
      | output = int t|input| dt
      mask Display:
      | disp('ITAE')
      | port_label('input',1,'e')
      | port_label('output',1,'itae')
  ITSE : Subsystem
      mask help:
      | ITAE performance index
      |
      | output = int t|input| dt
      mask Display:
      | disp('ITSE')
      | port_label('input',1,'e')
      | port_label('output',1,'itse')
  Subsystem1 : Subsystem
  Subsystem2 : Subsystem
  Subsystem3 : Subsystem
  Subsystem5 : Subsystem
  To File2 : ToFile  Filename=IAE_ACE_PI_5  MatrixName=IAE_ACE_PI_5
  To File28 : ToFile  Filename=ITAE_ACE_PI_5  MatrixName=ITAE_ACE_PI_5
  To File29 : ToFile  Filename=ISE_ACE_PI_5  MatrixName=ISE_ACE_PI_5
  To File30 : ToFile  Filename=ITSE_ACE_PI_5  MatrixName=ITSE_ACE_PI_5
  wires:
  ITAE5/1(Out1) -> Subsystem5/1(In1)
  ISE/1(Out1) -> Subsystem1/1(In1)
  Subsystem5/1(DP1) -> To File28/1
  In1/1 -> IAE/1(In1), ISE/1(In1), ITSE/1(In1), ITAE5/1(In1)
  IAE/1(Out1) -> Subsystem2/1(In1)
  Subsystem1/1(Out1) -> To File29/1
  Subsystem2/1(Out1) -> To File2/1
  ITSE/1(Out1) -> Subsystem3/1(In1)
  Subsystem3/1(Out1) -> To File30/1

== system PI_PSO/AREA 6/Performance Indices ==
  In1 : Inport
  IAE : Subsystem
      mask help:
      | IAE performacne index
      |
      | output = int |input| dt
      mask Display:
      | disp('IAE')
      | port_label('input',1,'e')
      | port_label('output',1,'iae')
  ISE : Subsystem
      mask help:
      | ISE performance index
      |
      | output = int (input)^2 dt
      mask Display:
      | disp('ISE')
      | port_label('input',1,'e')
      | port_label('output',1,'ise')
  ITAE6 : Subsystem
      mask help:
      | ITAE performance index
      |
      | output = int t|input| dt
      mask Display:
      | disp('ITAE')
      | port_label('input',1,'e')
      | port_label('output',1,'itae')
  ITSE : Subsystem
      mask help:
      | ITAE performance index
      |
      | output = int t|input| dt
      mask Display:
      | disp('ITSE')
      | port_label('input',1,'e')
      | port_label('output',1,'itse')
  Subsystem1 : Subsystem
  Subsystem2 : Subsystem
  Subsystem5 : Subsystem
  Subsystem6 : Subsystem
  To File27 : ToFile  Filename=IAE_ACE_PI_6  MatrixName=IAE_ACE_PI_6
  To File29 : ToFile  Filename=ISE_ACE_PI_6  MatrixName=ISE_ACE_PI_6
  To File30 : ToFile  Filename=ITSE_ACE_PI_6  MatrixName=ITSE_ACE_PI_6
  To File34 : ToFile  Filename=ITAE_ACE_PI_6  MatrixName=ITAE_ACE_PI_6
  wires:
  IAE/1(Out1) -> Subsystem2/1(In1)
  In1/1 -> IAE/1(In1), ITSE/1(In1), ISE/1(In1), ITAE6/1(In1)
  Subsystem2/1(Out1) -> To File27/1
  ITSE/1(Out1) -> Subsystem5/1(In1)
  Subsystem6/1(DP1) -> To File34/1
  ITAE6/1(Out1) -> Subsystem6/1(In1)
  Subsystem5/1(Out1) -> To File30/1
  Subsystem1/1(Out1) -> To File29/1
  ISE/1(Out1) -> Subsystem1/1(In1)

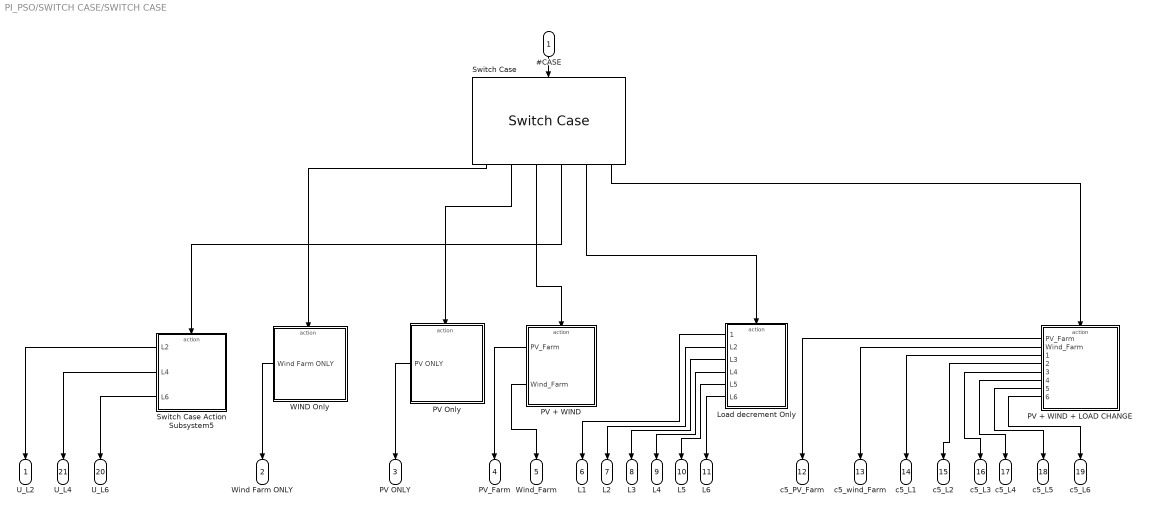
== system PI_PSO/SWITCH CASE/SWITCH CASE ==
  #CASE : Inport
  Load decrement Only : Subsystem  TreatAsAtomicUnit=on
  "PV + WIND " : Subsystem  TreatAsAtomicUnit=on
  PV + WIND + LOAD CHANGE : Subsystem  TreatAsAtomicUnit=on
  PV Only : Subsystem  TreatAsAtomicUnit=on
  Switch Case : SwitchCase  CaseConditions={0,1,2,3,4,5}  ShowDefaultCase=off
  Switch Case Action Subsystem5 : Subsystem  TreatAsAtomicUnit=on
  WIND Only : Subsystem  TreatAsAtomicUnit=on
  U_L2 : Outport
  "Wind Farm ONLY " : Outport  Port=2
  "PV ONLY " : Outport  Port=3
  "PV_Farm " : Outport  Port=4
  "Wind_Farm " : Outport  Port=5
  "L1 " : Outport  Port=6
  "L2 " : Outport  Port=7
  "L3 " : Outport  Port=8
  "L4 " : Outport  Port=9
  "L5 " : Outport  Port=10
  "L6 " : Outport  Port=11
  c5_PV_Farm : Outport  Port=12
  c5_wind_Farm : Outport  Port=13
  c5_L1 : Outport  Port=14
  c5_L2 : Outport  Port=15
  "c5_L3 " : Outport  Port=16
  c5_L4 : Outport  Port=17
  c5_L5 : Outport  Port=18
  c5_L6 : Outport  Port=19
  U_L6 : Outport  Port=20
  U_L4 : Outport  Port=21
  wires:
  PV + WIND + LOAD CHANGE/4("2 ") -> c5_L2/1
  PV + WIND + LOAD CHANGE/5("3 ") -> "c5_L3 "/1
  PV + WIND + LOAD CHANGE/2("Wind_Farm ") -> c5_wind_Farm/1
  PV + WIND + LOAD CHANGE/1("PV_Farm ") -> c5_PV_Farm/1
  PV + WIND + LOAD CHANGE/3("1 ") -> c5_L1/1
  #CASE/1 -> Switch Case/1
  "PV + WIND "/2("Wind_Farm ") -> "Wind_Farm "/1
  "PV + WIND "/1("PV_Farm ") -> "PV_Farm "/1
  PV Only/1("PV ONLY ") -> "PV ONLY "/1
  WIND Only/1("Wind Farm ONLY ") -> "Wind Farm ONLY "/1
  Switch Case/5 -> Load decrement Only/Action
  Switch Case/6 -> PV + WIND + LOAD CHANGE/Action
  Load decrement Only/1(" ") -> "L1 "/1
  Load decrement Only/2("L2 ") -> "L2 "/1
  Load decrement Only/3("L3 ") -> "L3 "/1
  Load decrement Only/4("L4 ") -> "L4 "/1
  Load decrement Only/5("L5 ") -> "L5 "/1
  Load decrement Only/6("L6 ") -> "L6 "/1
  PV + WIND + LOAD CHANGE/6(4) -> c5_L4/1
  PV + WIND + LOAD CHANGE/7("5 ") -> c5_L5/1
  PV + WIND + LOAD CHANGE/8("6 ") -> c5_L6/1
  Switch Case Action Subsystem5/1("L2 ") -> U_L2/1
  Switch Case Action Subsystem5/2("L4 ") -> U_L4/1
  Switch Case Action Subsystem5/3("L6 ") -> U_L6/1
  Switch Case/4 -> Switch Case Action Subsystem5/Action
  Switch Case/3 -> "PV + WIND "/Action
  Switch Case/1 -> WIND Only/Action
  Switch Case/2 -> PV Only/Action

== system PI_PSO/AREA 1/Performance Indices/IAE ==
  In1 : Inport
  Abs : Abs
  Discrete-Time Integrator : DiscreteIntegrator  gainval=1  SampleTime=-1  ICPrevOutput=DiscIntNeverNeededParam  ICPrevScaledInput=DiscIntNeverNeededParam
  Out1 : Outport
  wires:
  Abs/1 -> Discrete-Time Integrator/1
  Discrete-Time Integrator/1 -> Out1/1
  In1/1 -> Abs/1

== system PI_PSO/AREA 1/Performance Indices/ISE ==
  In1 : Inport
  Discrete-Time Integrator : DiscreteIntegrator  gainval=1  SampleTime=-1  ICPrevOutput=DiscIntNeverNeededParam  ICPrevScaledInput=DiscIntNeverNeededParam
  Math Function : Math  Operator=square  SignedPower=on  SaturateOnIntegerOverflow=on
  Out1 : Outport
  wires:
  In1/1 -> Math Function/1
  Discrete-Time Integrator/1 -> Out1/1
  Math Function/1 -> Discrete-Time Integrator/1

== system PI_PSO/AREA 1/Performance Indices/ITAE1 ==
  In1 : Inport
  Abs : Abs
  Clock : Clock
  Discrete-Time Integrator : DiscreteIntegrator  gainval=1  SampleTime=-1  ICPrevOutput=DiscIntNeverNeededParam  ICPrevScaledInput=DiscIntNeverNeededParam
  Divide : Product  Inputs=**
  Out1 : Outport
  wires:
  Clock/1 -> Divide/2
  Abs/1 -> Divide/1
  Divide/1 -> Discrete-Time Integrator/1
  In1/1 -> Abs/1
  Discrete-Time Integrator/1 -> Out1/1

== system PI_PSO/AREA 1/Performance Indices/ITSE ==
  In1 : Inport
  Clock : Clock
  Discrete-Time Integrator : DiscreteIntegrator  gainval=1  SampleTime=-1  ICPrevOutput=DiscIntNeverNeededParam  ICPrevScaledInput=DiscIntNeverNeededParam
  Divide : Product  Inputs=**
  Math Function : Math  Operator=square  SignedPower=on  SaturateOnIntegerOverflow=on
  Out1 : Outport
  wires:
  Discrete-Time Integrator/1 -> Out1/1
  In1/1 -> Math Function/1
  Divide/1 -> Discrete-Time Integrator/1
  Math Function/1 -> Divide/1
  Clock/1 -> Divide/2

== system PI_PSO/AREA 1/Performance Indices/Subsystem1 ==
  In1 : Inport
  Id_ref step : powerlib_extras/Control  Blocks/Timer  t=[0 1]  e=[0 1]
      settings: SourceProductBaseCode=PS
  Prod : Product  InputSameDT=on  SaturateOnIntegerOverflow=on  OutDataTypeStr=Inherit: Same as first input
  Out1 : Outport
  wires:
  Id_ref step/1 -> Prod/2
  In1/1 -> Prod/1
  Prod/1 -> Out1/1

== system PI_PSO/AREA 1/Performance Indices/Subsystem2 ==
  In1 : Inport
  Id_ref step : powerlib_extras/Control  Blocks/Timer  t=[0 1]  e=[0 1]
      settings: SourceProductBaseCode=PS
  Prod : Product  InputSameDT=on  SaturateOnIntegerOverflow=on  OutDataTypeStr=Inherit: Same as first input
  Out1 : Outport
  wires:
  Prod/1 -> Out1/1
  In1/1 -> Prod/1
  Id_ref step/1 -> Prod/2

== system PI_PSO/AREA 1/Performance Indices/Subsystem4 ==
  In1 : Inport
  Id_ref step : powerlib_extras/Control  Blocks/Timer  t=[0 1]  e=[0 1]
      settings: SourceProductBaseCode=PS
  Prod : Product  InputSameDT=on  SaturateOnIntegerOverflow=on  OutDataTypeStr=Inherit: Same as first input
  DP1 : Outport
  wires:
  Id_ref step/1 -> Prod/2
  In1/1 -> Prod/1
  Prod/1 -> DP1/1

== system PI_PSO/AREA 1/Performance Indices/Subsystem5 ==
  In1 : Inport
  Id_ref step : powerlib_extras/Control  Blocks/Timer  t=[0 1]  e=[0 1]
      settings: SourceProductBaseCode=PS
  Prod : Product  InputSameDT=on  SaturateOnIntegerOverflow=on  OutDataTypeStr=Inherit: Same as first input
  Out1 : Outport
  wires:
  Prod/1 -> Out1/1
  In1/1 -> Prod/1
  Id_ref step/1 -> Prod/2

== system PI_PSO/AREA 2/Performance Indices/IAE ==
  In1 : Inport
  Abs : Abs
  Discrete-Time Integrator : DiscreteIntegrator  gainval=1  SampleTime=-1  ICPrevOutput=DiscIntNeverNeededParam  ICPrevScaledInput=DiscIntNeverNeededParam
  Out1 : Outport
  wires:
  Abs/1 -> Discrete-Time Integrator/1
  Discrete-Time Integrator/1 -> Out1/1
  In1/1 -> Abs/1

== system PI_PSO/AREA 2/Performance Indices/ISE ==
  In1 : Inport
  Discrete-Time Integrator : DiscreteIntegrator  gainval=1  SampleTime=-1  ICPrevOutput=DiscIntNeverNeededParam  ICPrevScaledInput=DiscIntNeverNeededParam
  Math Function : Math  Operator=square  SignedPower=on  SaturateOnIntegerOverflow=on
  Out1 : Outport
  wires:
  In1/1 -> Math Function/1
  Discrete-Time Integrator/1 -> Out1/1
  Math Function/1 -> Discrete-Time Integrator/1

== system PI_PSO/AREA 2/Performance Indices/ITAE1 ==
  In1 : Inport
  Abs : Abs
  Clock : Clock
  Discrete-Time Integrator : DiscreteIntegrator  gainval=1  SampleTime=-1  ICPrevOutput=DiscIntNeverNeededParam  ICPrevScaledInput=DiscIntNeverNeededParam
  Divide : Product  Inputs=**
  Out1 : Outport
  wires:
  Clock/1 -> Divide/2
  Abs/1 -> Divide/1
  Divide/1 -> Discrete-Time Integrator/1
  In1/1 -> Abs/1
  Discrete-Time Integrator/1 -> Out1/1
